simulink model "chapter5"  (R2018a)
settings: Solver=VariableStepAuto  StartTime=0.0  StopTime=60  RelTol=1e-3
values from neighbouring files (symbols this model uses):
  C = [cs1       ,0        ,0        ,-cs1                   ,0              ,L1*cs1                       ,0 ... (first row only)    [vibs_project.m]
  K = [kt1+ks1,0       ,0       ,-ks1                  ,0                      ,L1*ks1                        ,0 ... (first row only)    [vibs_project.m]
  kt1 = 847000,kt2=2000000,kt3=2000000,ks1=300000,ks2=967430,ks3=155800,ks4=20000000    [vibs_project.m]
  M = [m1 ,0 ,0 ,0 ,0 ,0 ,0 ... (first row only)    [vibs_project.m]
  t1 = 0    [vibs_project.m]
  t2 = t1+(L1+L2)/V    [vibs_project.m]
  t3 = t2+(L5+L4+L3-L2)/V    [vibs_project.m]
  t_Y = L_Y/V    (= 0.09)    [vibs_project.m]
  Y = 0.1    [vibs_project.m]
settings Model: Creator=Toshiba  LastModifiedBy=Toshiba

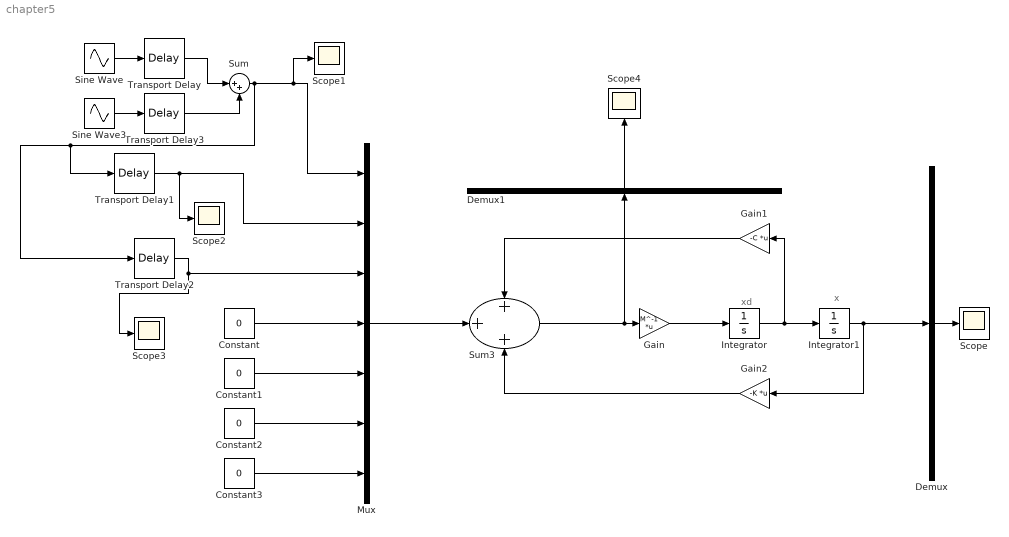
== system chapter5 ==
  note: x
  note: xd
  Constant{,1..3} (4 alike) : Constant  Value=0
  Demux : Demux  Outputs=7
  Demux1 : Demux  Outputs=7
  Gain : Gain  Gain=M^-1  Multiplication=Matrix(K*u)
  Gain1 : Gain  Gain=-C  Multiplication=Matrix(K*u)
  Gain2 : Gain  Gain=-K  Multiplication=Matrix(K*u)
  Integrator : Integrator
  Integrator1 : Integrator
  Mux : Mux  Inputs=7
  Scope{,1..4} (5 alike) : Scope
  Sine Wave : Sin  Amplitude=Y*kt1  Frequency=pi/t_Y  SampleTime=0
  Sine Wave3 : Sin  Amplitude=Y*kt1  Frequency=pi/t_Y  SampleTime=0
  Sum : Sum  Inputs=|++
  Sum3 : Sum  Inputs=+++
  Transport Delay : TransportDelay  DelayTime=t1
  Transport Delay1 : TransportDelay  DelayTime=t2
  Transport Delay2 : TransportDelay  DelayTime=t3
  Transport Delay3 : TransportDelay  DelayTime=t1+t_Y
  wires:
  Transport Delay1/1 -> Scope2/1, Mux/2
  Gain/1 -> Integrator/1
  Sum3/1 -> Demux1/1, Gain/1
  Constant2/1 -> Mux/6
  Mux/1 -> Sum3/2
  Constant1/1 -> Mux/5
  Integrator/1 -> Gain1/1, Integrator1/1
  Integrator1/1 -> Demux/1, Gain2/1
  Constant3/1 -> Mux/7
  Gain2/1 -> Sum3/3
  Constant/1 -> Mux/4
  Gain1/1 -> Sum3/1
  Demux/4 -> Scope/1
  Sine Wave/1 -> Transport Delay/1
  Sine Wave3/1 -> Transport Delay3/1
  Transport Delay/1 -> Sum/1
  Transport Delay3/1 -> Sum/2
  Sum/1 -> Transport Delay2/1, Transport Delay1/1, Scope1/1, Mux/1
  Transport Delay2/1 -> Mux/3, Scope3/1
  Demux1/4 -> Scope4/1
